simulink model "ZRM"  (R2021b)
settings: Solver=ode8  StartTime=0.0  StopTime=10.0  RelTol=1e-3
model workspace (MAT data in the model file):
  A = Simulink.Parameter
  A.Value = [0  1; 0  0]
  A.DataType = 'auto'
  A.Complexity = 'real'
  A.Dimensions = [2 2]
  B = Simulink.Parameter
  B.Value = 0.3
  B.DataType = 'auto'
  B.Complexity = 'real'
  B.Dimensions = [1 1]
  C = Simulink.Parameter
  C.Value = [1 0]
  C.DataType = 'auto'
  C.Complexity = 'real'
  C.Dimensions = [1 2]
  x0 = Simulink.Parameter
  x0.Value = 0.3
  x0.DataType = 'auto'
  x0.Complexity = 'real'
  x0.Dimensions = [1 1]
settings Model: ParameterArgumentNames=x0  Creator=Hoorsana  LastModifiedBy=Hoorsana

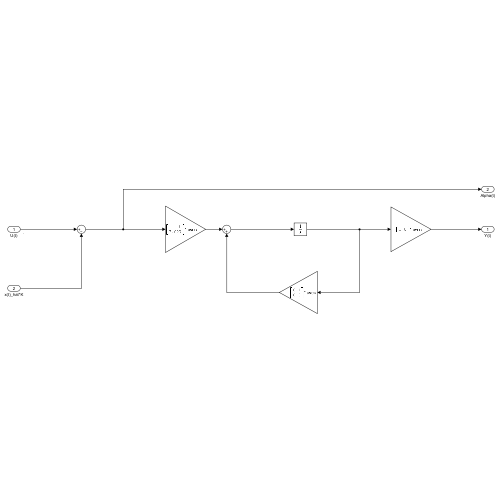
[thumbnail: Simulink's stored preview of the top-level diagram]
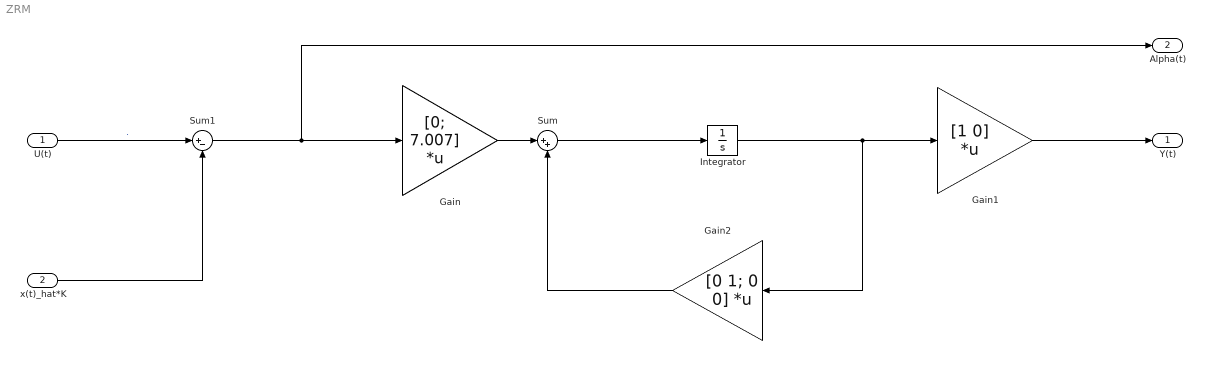
== system ZRM ==
  U(t) : Inport
  x(t)_hat*K : Inport  Port=2
  Gain : Gain  Gain=[0; 7.007]  Multiplication=Matrix(K*u) (u vector)
  Gain1 : Gain  Gain=[1 0]  Multiplication=Matrix(K*u) (u vector)
  Gain2 : Gain  Gain=[0 1; 0 0]  Multiplication=Matrix(K*u) (u vector)
  Integrator : Integrator  InitialCondition=x0
  Sum : Sum  Inputs=|++
  Sum1 : Sum  Inputs=|+-
  Y(t) : Outport  VectorParamsAs1DForOutWhenUnconnected=off
  Alpha(t) : Outport  Port=2  VectorParamsAs1DForOutWhenUnconnected=off
  wires:
  Gain1/1 -> Y(t)/1
  Integrator/1 -> Gain2/1, Gain1/1
  x(t)_hat*K/1 -> Sum1/2
  Gain/1 -> Sum/1
  U(t)/1 -> Sum1/1  "."
  Sum1/1 -> Alpha(t)/1, Gain/1
  Sum/1 -> Integrator/1
  Gain2/1 -> Sum/2
